simulink model "duty_cycle"  (Simulink 10.1)
settings: Solver=VariableStepDiscrete  StartTime=0.0  StopTime=2  RelTol=1e-3  EnableMultiTasking=on
libraries: speaker x1, amplitude_spectrum x1
settings Model: Creator=Administrator  LastModifiedBy=elezhan
settings DataIOCC: LimitDataPoints=on  SignalLoggingSaveFormat=ModelDataLogs
settings OptimizationCC: ExpressionDepthLimit=2147483647
settings DebuggingCC: SolverPrmCheckMsg=warning  FcnCallInpInsideContextMsg=warning  FrameProcessingCompatibilityMsg=none  StateNameClashWarn=warning
settings ConfigComp: CovSFcnEnable=off

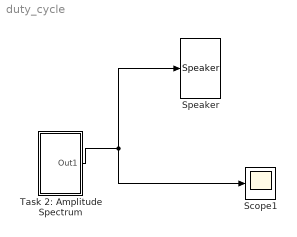
== system duty_cycle ==
  Scope1 : Scope
  Speaker : speaker/Speaker
  Task 2: Amplitude Spectrum : Subsystem  mask(Amplitude spectrum square waveforms.){tau=50}
      mask prompts: tau "Duty Cycle"
      mask help:
      | Input square waveform freqeuncy f =2k Hz and duty cycle tau.
      | tau is an integer number in the range of [10,90] meanig the duty cycel is tau%..
  wires:
  Task 2: Amplitude Spectrum/1(Out1) -> Scope1/1, Speaker/1

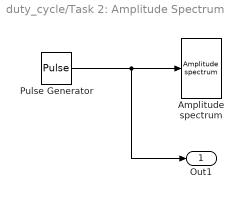
== system duty_cycle/Task 2: Amplitude Spectrum ==
  Amplitude spectrum : amplitude_spectrum/Amplitude spectrum
  Pulse Generator : DiscretePulseGenerator  PulseType=Time based  Period=1/2000  PulseWidth=tau
  Out1 : Outport  VectorParamsAs1DForOutWhenUnconnected=off
  wires:
  Pulse Generator/1 -> Out1/1, Amplitude spectrum/1
